simulink model "eqDiffLin"  (R2020a)
settings: Solver=ode1  StartTime=0.0  StopTime=10.0  RelTol=1e-3
settings Model: Creator=aless  LastModifiedBy=aless

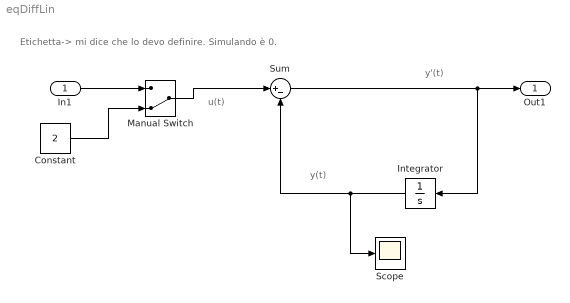
== system eqDiffLin ==
  note: y(t)
  note: u(t)
  note: Etichetta-> mi dice che lo devo definire. Simulando è 0.
  note: y'(t)
  In1 : Inport
  Constant : Constant  Value=2
  Integrator : Integrator  InitialCondition=1
  Manual Switch : ManualSwitch  CurrentSetting=0
  Scope : Scope
  Sum : Sum  Inputs=|+-
  Out1 : Outport
  wires:
  Sum/1 -> Integrator/1, Out1/1
  Integrator/1 -> Scope/1, Sum/2
  In1/1 -> Manual Switch/1
  Manual Switch/1 -> Sum/1
  Constant/1 -> Manual Switch/2
